simulink model "coupled_inductor_test"  (Simulink 7.4)
settings: Solver=ode45  StartTime=0.0  StopTime=10e-5  MaxStep=.001  RelTol=1e-4
StartFcn:
  | tic
StopFcn:
  | trun=toc
undefined symbols (not defined in the file or in its folder): Fs, magnitude
libraries: powerlib x16, dspindex x6, dsparch4 x5, dspsigops x3, dspsnks4 x2, dspbuff3 x2, dspxfrm3 x2, dsparch3 x2, dspmtrx3 x1, simulink x1
settings Model: Creator=Owner  LastModifiedBy=Dick
settings DataIOCC: SignalLoggingName=sigsOut
settings OptimizationCC: InlineInvariantSignals=on  InitFltsAndDblsToZero=on
settings DebuggingCC: SaveWithParameterizedLinksMsg=none  SignalResolutionControl=TryResolveAllWithWarning  SolverPrmCheckMsg=none  MultiTaskDSMMsg=warning  MultiTaskCondExecSysMsg=none  StrictBusMsg=None
settings HardwareCC: TargetUnknown=on
settings RTWCC: IncludeERTFirstTime=on
settings GRTTargetCC: TargetFcnLib=ansi_tfl_tmw.mat

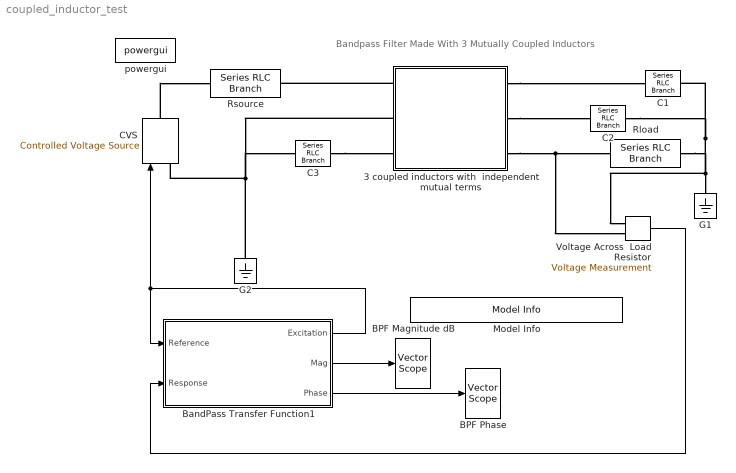
== system coupled_inductor_test ==
  note: Bandpass Filter Made With 3 Mutually Coupled Inductors
  3 coupled inductors with  independent mutual terms : Subsystem  mask{L1=1e-6, L2=1e-6, L3=1e-6, M12=0.1e-6, M23=0.1e-6, M13=1e-8}
      mask prompts: L1 "L1="; L2 "L2="; L3 "L3="; M12 "M12="; M23 "M23="; M13 "M13="
  BPF Magnitude dB : dspsnks4/Vector Scope  DialogController=dspdialog.VectorScope  DialogControllerArgs=DataTag0  ScopeProperties=on  Domain=Frequency  HorizSpan=1  DisplayProperties=off  AxisGrid=on  Memory=off  FrameNumber=on  AxisLegend=off  AxisZoom=off  OpenScopeAtSimStart=on  OpenScopeImmediately=off  FigPos=[38 401 372 236]  AxisProperties=off  XUnits=Hertz  XRange=[-Fs/2...Fs/2]  InheritXIncr=on  XIncr=2*Fs  XLabel=Time  XLimit=Auto  XMin=0  XMax=1  XStart=0  YUnits=dB  YLabel=dB  LineProperties=off  LineColors=[0 0 1]|[1 0 0]  XAxisParamsVer=6.9
      settings: YMin=-60  YMax=0
  BPF Phase : dspsnks4/Vector Scope  DialogController=dspdialog.VectorScope  DialogControllerArgs=DataTag1  ScopeProperties=on  Domain=Frequency  HorizSpan=1  DisplayProperties=off  AxisGrid=on  Memory=off  FrameNumber=on  AxisLegend=off  AxisZoom=off  OpenScopeAtSimStart=on  OpenScopeImmediately=off  FigPos=[37 115 372 236]  AxisProperties=off  XUnits=Hertz  XRange=[-Fs/2...Fs/2]  InheritXIncr=on  XIncr=2*Fs  XLabel=Time  XLimit=Auto  XMin=0  XMax=1  XStart=0  YUnits=Magnitude  YLabel=Degrees  LineProperties=off  LineColors=[0 0 1]|[1 0 0]  XAxisParamsVer=6.9
      settings: YMin=-253.502574206464  YMax=262.314910592616
  BandPass Transfer Function1 : Subsystem  Description=Spectrum Analyzer  mask{BW=40e6, Fc=100e6, NFFT=1024, Avg_fac=100}
      mask prompts: BW "Bandwidth"; Fc "Center Freq"; NFFT "FFT Length (power of 2)"; Avg_fac "Averaging Factor (>=1)"
  C1 : powerlib/Elements/Series RLC Branch  DialogController=POWERSYS.PowerSysDialog  PhysicalDomain=powersysdomain  SubClassName=unknown  LeftPortType=p1  RightPortType=p1  LConnTagsString=__new0  RConnTagsString=__new0  BranchType=C  Resistance=1.0  Inductance=1.0  SetiL0=off  InitialCurrent=0  Capacitance=2.5e-12  Setx0=off  InitialVoltage=0  Measurements=None
  C2 : powerlib/Elements/Series RLC Branch  DialogController=POWERSYS.PowerSysDialog  PhysicalDomain=powersysdomain  SubClassName=unknown  LeftPortType=p1  RightPortType=p1  LConnTagsString=__new0  RConnTagsString=__new0  BranchType=C  Resistance=1.0  Inductance=1.0  SetiL0=off  InitialCurrent=0  Capacitance=2.5e-12  Setx0=off  InitialVoltage=0  Measurements=None
  C3 : powerlib/Elements/Series RLC Branch  DialogController=POWERSYS.PowerSysDialog  PhysicalDomain=powersysdomain  SubClassName=unknown  LeftPortType=p1  RightPortType=p1  LConnTagsString=__new0  RConnTagsString=__new0  BranchType=C  Resistance=1.0  Inductance=1.0  SetiL0=off  InitialCurrent=0  Capacitance=2.5e-12  Setx0=off  InitialVoltage=0  Measurements=None
  CVS : powerlib/Electrical Sources/Controlled Voltage Source  Description=source block  DialogController=POWERSYS.PowerSysDialog  SystemSampleTime=-1  Initialize=on  Source_Type=AC  Amplitude=0  Phase=0  Frequency=0  Measurements=None
      settings: AttributesFormatString=\n
  G1 : powerlib/Elements/Ground  DialogController=POWERSYS.PowerSysDialog  PhysicalDomain=powersysdomain  SubClassName=unknown  LeftPortType=p1  RightPortType=p1  LConnTagsString=a
  G2 : powerlib/Elements/Ground  DialogController=POWERSYS.PowerSysDialog  PhysicalDomain=powersysdomain  SubClassName=unknown  LeftPortType=p1  RightPortType=p1  LConnTagsString=a
  Model Info : simulink/Model-Wide Utilities/Model Info  SystemSampleTime=-1  InitialBlockCM=None  BlockCM=None  Frame=on  DisplayStringWithTags=Copywrite 2005-2010 The MathWorks, Inc.  HorizontalTextAlignment=Center  LeftAlignmentValue=0.5  SourceBlockDiagram=coupled_inductor_test  TagMaxNumber=20
  Rload : powerlib/Elements/Series RLC Branch  DialogController=POWERSYS.PowerSysDialog  PhysicalDomain=powersysdomain  SubClassName=unknown  LeftPortType=p1  RightPortType=p1  LConnTagsString=__new0  RConnTagsString=__new0  BranchType=R  Resistance=50  Inductance=1.0  SetiL0=off  InitialCurrent=0  Capacitance=1.0  Setx0=off  InitialVoltage=0  Measurements=None
  Rsource : powerlib/Elements/Series RLC Branch  DialogController=POWERSYS.PowerSysDialog  PhysicalDomain=powersysdomain  SubClassName=unknown  LeftPortType=p1  RightPortType=p1  LConnTagsString=__new0  RConnTagsString=__new0  BranchType=R  Resistance=50  Inductance=1.0  SetiL0=off  InitialCurrent=0  Capacitance=1.0  Setx0=off  InitialVoltage=0  Measurements=None
  Voltage Across  Load Resistor : powerlib/Measurements/Voltage Measurement  Tag=PoWeRsYsTeMmEaSuReMeNt  DialogController=POWERSYS.PowerSysDialog  SystemSampleTime=-1  PhasorSimulation=off  OutputType=Magnitude  PSBequivalent=0
  powergui : powerlib/powergui  SystemSampleTime=-1  SimulationMode=Continuous  SampleTime=0  frequency=60  SPID=off  DisableSnubberDevices=off  DisableRonSwitches=off  DisableVfSwitches=off  SwTol=0  Interpol=off  frequencyindice=0  echomessages=off  HookPort=off  DisplayEquations=off  FunctionMessages=off  EnableUseOfTLC=off  x0status=blocks  RestoreLinks=warning  Frange=[0:2:500]  Ylog=off  Xlog=on  ShowGrid=off  save=off  variable=ZData  ZoomFFT=on  StartTime=0.0  cycles=1  DisplayStyle=1  fundamental=60  FreqAxis=off  MaxFrequency=1000  frequencyindicesteady=1  RmsSteady=1  display=off  Ts=0  methode=off
  wires:
  Voltage Across  Load Resistor/1 -> BandPass Transfer Function1/2(Response)
  BandPass Transfer Function1/1(Excitation) -> CVS/1, BandPass Transfer Function1/1(Reference)
  BandPass Transfer Function1/2(Mag) -> BPF Magnitude dB/1
  BandPass Transfer Function1/3(Phase) -> BPF Phase/1
  connections:
  3 coupled inductors with  independent mutual terms/LConn1 -- Rsource/RConn1
  CVS/RConn1 -- Rsource/LConn1
  C1/RConn1 -- C2/RConn1 -- Rload/RConn1 -- G1/LConn1 -- Voltage Across  Load Resistor/LConn1
  3 coupled inductors with  independent mutual terms/RConn3 -- Rload/LConn1 -- Voltage Across  Load Resistor/LConn2
  3 coupled inductors with  independent mutual terms/RConn2 -- C2/LConn1
  3 coupled inductors with  independent mutual terms/RConn1 -- C1/LConn1
  C3/RConn1 -- 3 coupled inductors with  independent mutual terms/LConn3
  G2/LConn1 -- 3 coupled inductors with  independent mutual terms/LConn2 -- C3/LConn1 -- CVS/LConn1

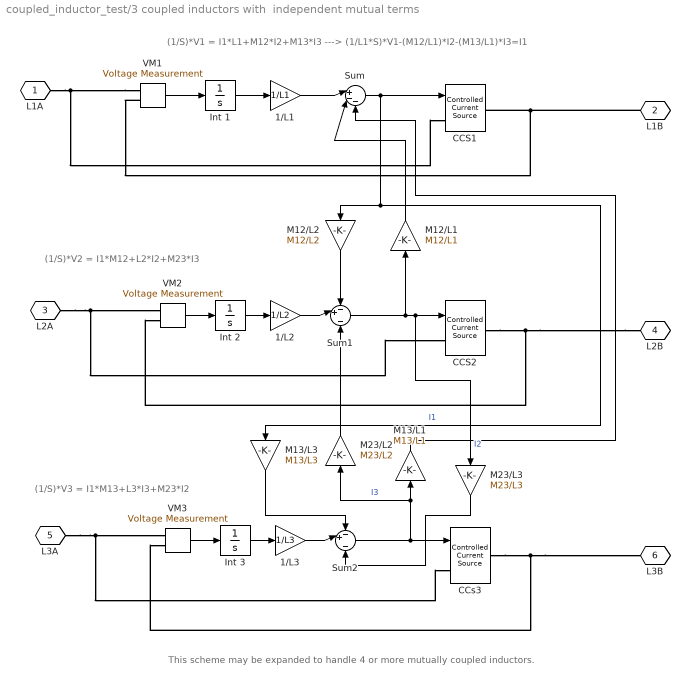
== system coupled_inductor_test/3 coupled inductors with  independent mutual terms ==
  note: (1/S)*V1 = I1*L1+M12*I2+M13*I3 ---> (1/L1*S)*V1-(M12/L1)*I2-(M13/L1)*I3=I1
  note: (1/S)*V2 = I1*M12+L2*I2+M23*I3
  note: (1/S)*V3 = I1*M13+L3*I3+M23*I2
  note: This scheme may be expanded to handle 4 or more mutually coupled inductors.
  1/L1 : Gain  Gain=1/L1  ParameterDataType=sfix(16)  ParameterScaling=2^0  OutDataType=sfix(16)  OutScaling=2^0  SaturateOnIntegerOverflow=on  OutDataTypeStr=Inherit: Same as input  ParamDataTypeStr=Inherit: Same as input
  1/L2 : Gain  Gain=1/L2  ParameterDataType=sfix(16)  ParameterScaling=2^0  OutDataType=sfix(16)  OutScaling=2^0  SaturateOnIntegerOverflow=on  OutDataTypeStr=Inherit: Same as input  ParamDataTypeStr=Inherit: Same as input
  1/L3 : Gain  Gain=1/L3  ParameterDataType=sfix(16)  ParameterScaling=2^0  OutDataType=sfix(16)  OutScaling=2^0  SaturateOnIntegerOverflow=on  OutDataTypeStr=Inherit: Same as input  ParamDataTypeStr=Inherit: Same as input
  CCS1 : powerlib/Electrical Sources/Controlled Current Source  Description=source block  DialogController=POWERSYS.PowerSysDialog  SystemSampleTime=-1  Initialize=off  Source_Type=AC  Amplitude=0  Phase=0  Frequency=0  Measurements=None
      settings: AttributesFormatString=\n
  CCS2 : powerlib/Electrical Sources/Controlled Current Source  Description=source block  DialogController=POWERSYS.PowerSysDialog  SystemSampleTime=-1  Initialize=off  Source_Type=AC  Amplitude=0  Phase=0  Frequency=0  Measurements=None
      settings: AttributesFormatString=\n
  CCs3 : powerlib/Electrical Sources/Controlled Current Source  Description=source block  DialogController=POWERSYS.PowerSysDialog  SystemSampleTime=-1  Initialize=off  Source_Type=AC  Amplitude=0  Phase=0  Frequency=0  Measurements=None
      settings: AttributesFormatString=\n
  Int 1 : Integrator
  Int 2 : Integrator
  Int 3 : Integrator
  M12/L1 : Gain  Gain=M12/L1  ParameterDataType=sfix(16)  ParameterScaling=2^0  OutDataType=sfix(16)  OutScaling=2^0  SaturateOnIntegerOverflow=on  OutDataTypeStr=Inherit: Same as input  ParamDataTypeStr=Inherit: Same as input
  M12/L2 : Gain  Gain=M12/L2  ParameterDataType=sfix(16)  ParameterScaling=2^0  OutDataType=sfix(16)  OutScaling=2^0  SaturateOnIntegerOverflow=on  OutDataTypeStr=Inherit: Same as input  ParamDataTypeStr=Inherit: Same as input
  M13/L1 : Gain  Gain=M13/L1  ParameterDataType=sfix(16)  ParameterScaling=2^0  OutDataType=sfix(16)  OutScaling=2^0  SaturateOnIntegerOverflow=on  OutDataTypeStr=Inherit: Same as input  ParamDataTypeStr=Inherit: Same as input
  M13/L3 : Gain  Gain=M13/L3  ParameterDataType=sfix(16)  ParameterScaling=2^0  OutDataType=sfix(16)  OutScaling=2^0  SaturateOnIntegerOverflow=on  OutDataTypeStr=Inherit: Same as input  ParamDataTypeStr=Inherit: Same as input
  M23/L2 : Gain  Gain=M23/L2  ParameterDataType=sfix(16)  ParameterScaling=2^0  OutDataType=sfix(16)  OutScaling=2^0  SaturateOnIntegerOverflow=on  OutDataTypeStr=Inherit: Same as input  ParamDataTypeStr=Inherit: Same as input
  M23/L3 : Gain  Gain=M23/L3  ParameterDataType=sfix(16)  ParameterScaling=2^0  OutDataType=sfix(16)  OutScaling=2^0  SaturateOnIntegerOverflow=on  OutDataTypeStr=Inherit: Same as input  ParamDataTypeStr=Inherit: Same as input
  Sum : Sum  Inputs=|+--  OutDataType=sfix(16)  OutScaling=2^0  SaturateOnIntegerOverflow=on
  Sum1 : Sum  Inputs=-+|-  OutDataType=sfix(16)  OutScaling=2^0  SaturateOnIntegerOverflow=on
  Sum2 : Sum  Inputs=-+|-  OutDataType=sfix(16)  OutScaling=2^0  SaturateOnIntegerOverflow=on
  VM1 : powerlib/Measurements/Voltage Measurement  Tag=PoWeRsYsTeMmEaSuReMeNt  DialogController=POWERSYS.PowerSysDialog  SystemSampleTime=-1  PhasorSimulation=off  OutputType=Magnitude  PSBequivalent=0
  VM2 : powerlib/Measurements/Voltage Measurement  Tag=PoWeRsYsTeMmEaSuReMeNt  DialogController=POWERSYS.PowerSysDialog  SystemSampleTime=-1  PhasorSimulation=off  OutputType=Magnitude  PSBequivalent=0
  VM3 : powerlib/Measurements/Voltage Measurement  Tag=PoWeRsYsTeMmEaSuReMeNt  DialogController=POWERSYS.PowerSysDialog  SystemSampleTime=-1  PhasorSimulation=off  OutputType=Magnitude  PSBequivalent=0
  L1A : PMIOPort  Tag=PMCPort  Port=1  Side=Left
  L1B : PMIOPort  Tag=PMCPort  Port=2  Side=Right
  L2A : PMIOPort  Tag=PMCPort  Port=3  Side=Left
  L2B : PMIOPort  Tag=PMCPort  Port=4  Side=Right
  L3A : PMIOPort  Tag=PMCPort  Port=5  Side=Left
  L3B : PMIOPort  Tag=PMCPort  Port=6  Side=Right
  wires:
  Int 1/1 -> 1/L1/1
  VM1/1 -> Int 1/1
  Int 2/1 -> 1/L2/1
  VM2/1 -> Int 2/1
  1/L1/1 -> Sum/1
  Sum/1 -> CCS1/1, M12/L2/1, M13/L3/1  "I1"
  Sum1/1 -> M12/L1/1, CCS2/1, M23/L3/1  "I2"
  1/L2/1 -> Sum1/2
  M12/L1/1 -> Sum/2
  M12/L2/1 -> Sum1/1
  Int 3/1 -> 1/L3/1
  VM3/1 -> Int 3/1
  Sum2/1 -> CCs3/1, M13/L1/1, M23/L2/1  "I3"
  1/L3/1 -> Sum2/2
  M13/L1/1 -> Sum/3
  M23/L2/1 -> Sum1/3
  M13/L3/1 -> Sum2/1
  M23/L3/1 -> Sum2/3
  connections:
  VM1/LConn1 -- L1A/RConn1 -- CCS1/LConn1
  VM1/LConn2 -- CCS1/RConn1 -- L1B/RConn1
  L2A/RConn1 -- VM2/LConn1 -- CCS2/LConn1
  L2B/RConn1 -- CCS2/RConn1 -- VM2/LConn2
  CCs3/LConn1 -- L3A/RConn1 -- VM3/LConn1
  VM3/LConn2 -- L3B/RConn1 -- CCs3/RConn1

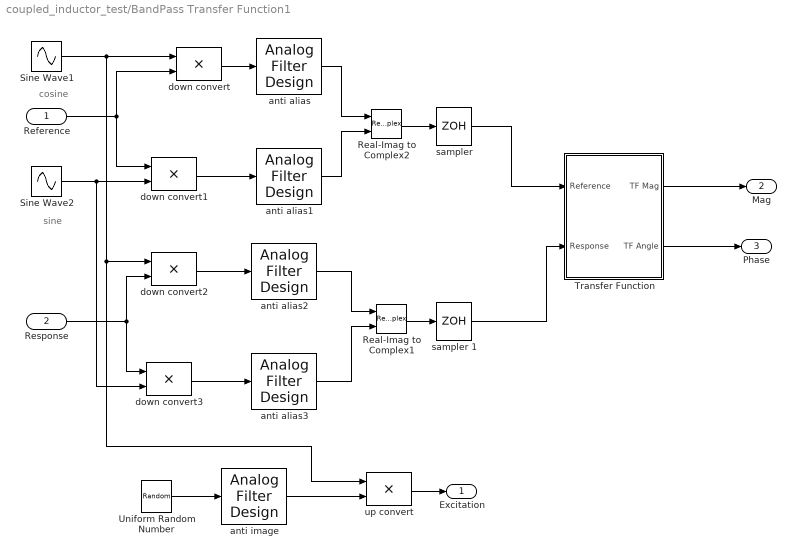
== system coupled_inductor_test/BandPass Transfer Function1 ==
  note: sine
  note: cosine
  Reference : Inport  OutDataType=sfix(16)  OutScaling=2^0
  Response : Inport  Port=2  OutDataType=sfix(16)  OutScaling=2^0
  Real-Imag to Complex1 : RealImagToComplex
  Real-Imag to Complex2 : RealImagToComplex
  Sine Wave1 : Sin  Amplitude=1  Bias=0  Frequency=2*pi*(Fc)  Phase=-pi/2  Samples=10  SampleTime=0  Offset=0
  Sine Wave2 : Sin  Amplitude=1  Bias=0  Frequency=2*pi*(Fc)  Phase=0  Samples=10  SampleTime=0  Offset=0
  "Transfer Function " : Subsystem  mask{NFFT=NFFT, Navg=Avg_fac, pcnt=100/1.28, unwrap_flag=on}
      mask prompts: NFFT "FFT length (power of 2):"; Navg "Spectral Averaging Factor (>=1):"; pcnt "Percentage of  Alias Free Data  (<=100)"; unwrap_flag "Unwrap Phase"
      mask Display: disp('Transfer Function \n Estimation (v2.0) ')
  Uniform Random Number : UniformRandomNumber  SampleTime=1/(2.56*BW)
  anti alias{,1..3} (4 alike) : dsparch4/Analog Filter Design  method=Elliptic  filttype=Lowpass  N=8  Wlo=BW*pi  Whi=80  Rp=2  Rs=100
  anti image : dsparch4/Analog Filter Design  method=Elliptic  filttype=Lowpass  N=9  Wlo=BW*pi  Whi=80  Rp=2  Rs=100
  down convert{,1..3} (4 alike) : Product  OutDataType=sfix(16)  OutScaling=2^0  SaturateOnIntegerOverflow=on  InputSameDT=on  OutDataTypeStr=Inherit: Same as first input
  "sampler " : ZeroOrderHold  SampleTime=1/(1.28*BW)
  sampler 1 : ZeroOrderHold  SampleTime=1/(1.28*BW)
  up convert : Product  OutDataType=sfix(16)  OutScaling=2^0  SaturateOnIntegerOverflow=on  InputSameDT=on  OutDataTypeStr=Inherit: Same as first input
  Excitation : Outport  OutDataType=sfix(16)  OutScaling=2^0
  Mag : Outport  Port=2  OutDataType=sfix(16)  OutScaling=2^0
  Phase : Outport  Port=3  OutDataType=sfix(16)  OutScaling=2^0
  wires:
  anti image/1 -> up convert/2
  down convert1/1 -> anti alias1/1
  sampler 1/1 -> "Transfer Function "/2(Response)
  "sampler "/1 -> "Transfer Function "/1(Reference)
  Real-Imag to Complex2/1 -> "sampler "/1
  anti alias1/1 -> Real-Imag to Complex2/2
  anti alias/1 -> Real-Imag to Complex2/1
  "Transfer Function "/2(TF Angle) -> Phase/1
  "Transfer Function "/1(TF Mag) -> Mag/1
  up convert/1 -> Excitation/1
  Uniform Random Number/1 -> anti image/1
  Real-Imag to Complex1/1 -> sampler 1/1
  down convert3/1 -> anti alias3/1
  anti alias3/1 -> Real-Imag to Complex1/2
  anti alias2/1 -> Real-Imag to Complex1/1
  down convert2/1 -> anti alias2/1
  Response/1 -> down convert2/2, down convert3/1
  Sine Wave2/1 -> down convert3/2, down convert1/2
  Sine Wave1/1 -> up convert/1, down convert2/1, down convert/1
  down convert/1 -> anti alias/1
  Reference/1 -> down convert1/1, down convert/2

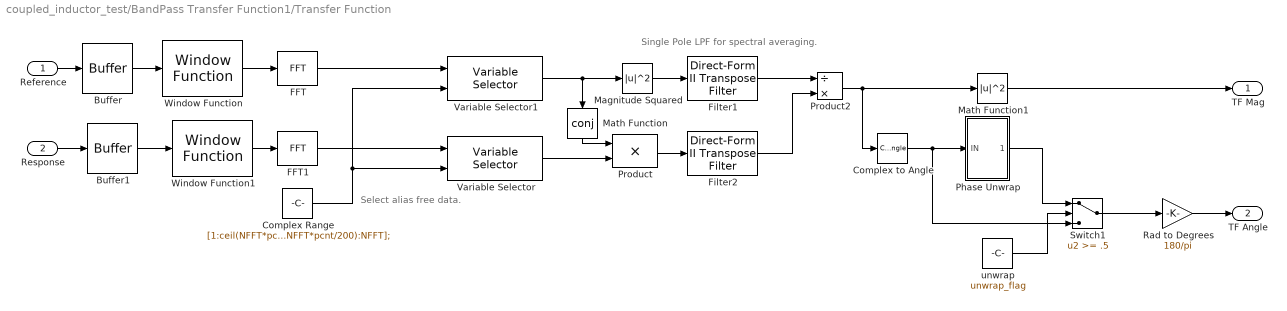
== system coupled_inductor_test/BandPass Transfer Function1/Transfer Function  ==
  note: Select alias free data.
  note: Single Pole LPF for spectral averaging.
  Reference : Inport  OutDataType=sfix(16)  OutScaling=2^0
  Response : Inport  Port=2  OutDataType=sfix(16)  OutScaling=2^0
  Buffer : dspbuff3/Buffer  N=NFFT  V=0  ic=0
  Buffer1 : dspbuff3/Buffer  N=NFFT  V=0  ic=0
  Complex Range : Constant  Value=[1:ceil(NFFT*pcnt/200),ceil(1+NFFT-NFFT*pcnt/200):NFFT];  OutDataType=sfix(16)  OutScaling=2^0
  Complex to Angle : ComplexToMagnitudeAngle  Output=Angle
  FFT : dspxfrm3/FFT  DialogController=dspDDGCreate  DialogControllerArgs=DataTag2  CompMethod=Table lookup  TableOpt=NEW  TableOptActive=Speed  BitRevOrder=off  InheritFFTLength=on  FFTLength=64  SkipNorm=on  firstCoeffMode=Specify word length  firstCoeffWordLength=16  firstCoeffFracLength=15  roundingMode=Floor  overflowMode=off
  FFT1 : dspxfrm3/FFT  DialogController=dspDDGCreate  DialogControllerArgs=DataTag3  CompMethod=Table lookup  TableOpt=NEW  TableOptActive=Speed  BitRevOrder=off  InheritFFTLength=on  FFTLength=64  SkipNorm=on  firstCoeffMode=User-defined  firstCoeffWordLength=16  firstCoeffFracLength=15  roundingMode=Floor  overflowMode=off
  Filter1 : dsparch3/Direct-Form II Transpose Filter  num=1  den=[Navg -(Navg-1)]  ic=eps
  Filter2 : dsparch3/Direct-Form II Transpose Filter  num=1  den=[Navg -(Navg-1)]  ic=eps
  Magnitude Squared : Math  Operator=magnitude^2  OutDataType=sfix(16)  OutScaling=2^0  SaturateOnIntegerOverflow=on
  Math Function : Math  Operator=conj  OutDataType=sfix(16)  OutScaling=2^0  SaturateOnIntegerOverflow=on
  Math Function1 : Math  Operator=magnitude^2  OutDataType=sfix(16)  OutScaling=2^0  SaturateOnIntegerOverflow=on
  Phase Unwrap : Subsystem
  Product : Product  OutDataType=sfix(16)  OutScaling=2^0  SaturateOnIntegerOverflow=on  InputSameDT=on  OutDataTypeStr=Inherit: Same as first input
  Product2 : Product  Inputs=/*  OutDataType=sfix(16)  OutScaling=2^0  SaturateOnIntegerOverflow=on  InputSameDT=on  OutDataTypeStr=Inherit: Same as first input
  Rad to Degrees : Gain  Gain=180/pi  ParameterDataType=sfix(16)  ParameterScaling=2^0  OutDataType=sfix(16)  OutScaling=2^0
  Switch1 : Switch  Threshold=.5
  Variable Selector : dspindex/Variable Selector  NumInputs=1  rowsOrCols=Rows  IdxMode=Variable  Elements=[1 3]  ZerOneIdxMode=One-based  errmode=Clip Index  FillMode=on  FillValues=0
  Variable Selector1 : dspindex/Variable Selector  NumInputs=1  rowsOrCols=Rows  IdxMode=Variable  Elements=[1 3]  ZerOneIdxMode=One-based  errmode=Clip Index  FillMode=on  FillValues=0
  Window Function : dspsigops/Window Function  DialogController=dspDDGCreate  DialogControllerArgs=DataTag5  winmode=Apply window to input  wintype=Hann  sampmode=Continuous  samptime=1  N=64  Rs=50  beta=10  winsamp=Periodic  UserWindow=hamming  OptParams=off  UserParams={'symmetric'}  dataType=double  isSigned=on  wordLen=16  udDataType=sfix(16)  fracBitsMode=Best precision  numFracBits=15  roundingMode=Floor  overflowMode=off  numSidelobes=4  sidelobeLevel=-30
  Window Function1 : dspsigops/Window Function  DialogController=dspDDGCreate  DialogControllerArgs=DataTag6  winmode=Apply window to input  wintype=Hann  sampmode=Continuous  samptime=1  N=64  Rs=50  beta=10  winsamp=Periodic  UserWindow=hamming  OptParams=off  UserParams={'symmetric'}  dataType=double  isSigned=on  wordLen=16  udDataType=sfix(16)  fracBitsMode=Best precision  numFracBits=15  roundingMode=Floor  overflowMode=off  numSidelobes=4  sidelobeLevel=-30
  unwrap : Constant  Value=unwrap_flag  OutDataType=sfix(16)  OutScaling=2^0
  TF Mag : Outport  OutDataType=sfix(16)  OutScaling=2^0
  TF Angle : Outport  Port=2  OutDataType=sfix(16)  OutScaling=2^0
  wires:
  Phase Unwrap/1(Out1) -> Switch1/1
  unwrap/1 -> Switch1/2
  Switch1/1 -> Rad to Degrees/1
  Variable Selector1/1 -> Math Function/1, Magnitude Squared/1
  Variable Selector/1 -> Product/2
  Product2/1 -> Math Function1/1, Complex to Angle/1
  Buffer1/1 -> Window Function1/1
  Buffer/1 -> Window Function/1
  Filter2/1 -> Product2/2
  Filter1/1 -> Product2/1
  Window Function1/1 -> FFT1/1
  Window Function/1 -> FFT/1
  Math Function1/1 -> TF Mag/1
  FFT/1 -> Variable Selector1/1
  Magnitude Squared/1 -> Filter1/1
  Math Function/1 -> Product/1
  FFT1/1 -> Variable Selector/1
  Product/1 -> Filter2/1
  Reference/1 -> Buffer/1
  Response/1 -> Buffer1/1
  Rad to Degrees/1 -> TF Angle/1
  Complex to Angle/1 -> Phase Unwrap/1(IN), Switch1/3
  Complex Range/1 -> Variable Selector1/2, Variable Selector/2

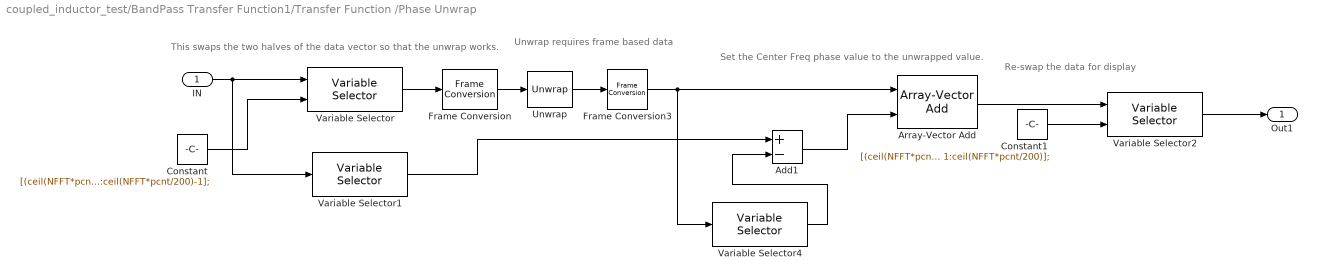
== system coupled_inductor_test/BandPass Transfer Function1/Transfer Function /Phase Unwrap ==
  note: Unwrap requires frame based data
  note: Re-swap the data for display
  note: Set the Center Freq phase value to the unwrapped value.
  note: This swaps the two halves of the data vector
      | so that the unwrap works.
  IN : Inport  OutDataType=sfix(16)  OutScaling=2^0
  Add1 : Sum  Inputs=+-  OutDataType=sfix(16)  OutScaling=2^-10
  Array-Vector Add : dspmtrx3/Array-Vector Add  DialogController=dspDDGCreate  DialogControllerArgs=DataTag4  Dimension=2  V_Source=Input port  V_VectFromMask=[0.5 0.25]  firstCoeffDataTypeStr=Inherit: Same word length as input  firstCoeffLastDataTypeStr=Inherit: Same word length as input  firstCoeffMin=[]  firstCoeffMax=[]  outputDataTypeStr=Inherit: Same as accumulator  outputLastDataTypeStr=Inherit: Same as accumulator  outputMin=[]  outputMax=[]  roundingMode=Floor  overflowMode=off
  Constant : Constant  Value=[(ceil(NFFT*pcnt/200)):ceil(NFFT*pcnt/100) 1:ceil(NFFT*pcnt/200)-1];  OutDataType=sfix(16)  OutScaling=2^0
  Constant1 : Constant  Value=[(ceil(NFFT*pcnt/200)+1):ceil(NFFT*pcnt/100) 1:ceil(NFFT*pcnt/200)];  OutDataType=sfix(16)  OutScaling=2^0
  Frame Conversion : FrameConversion
  Frame Conversion3 : FrameConversion  OutFrame=Sample-based
  Unwrap : dspsigops/Unwrap  running=on  tol=pi
  Variable Selector : dspindex/Variable Selector  NumInputs=1  rowsOrCols=Rows  IdxMode=Variable  Elements=[1 3]  ZerOneIdxMode=One-based  errmode=Clip Index  FillMode=on  FillValues=0
  Variable Selector1 : dspindex/Variable Selector  NumInputs=1  rowsOrCols=Rows  IdxMode=Fixed  Elements=[1]  ZerOneIdxMode=One-based  errmode=Clip Index  FillMode=on  FillValues=0
  Variable Selector2 : dspindex/Variable Selector  NumInputs=1  rowsOrCols=Rows  IdxMode=Variable  Elements=[1 3]  ZerOneIdxMode=One-based  errmode=Clip Index  FillMode=on  FillValues=0
  Variable Selector4 : dspindex/Variable Selector  NumInputs=1  rowsOrCols=Rows  IdxMode=Fixed  Elements=length([(ceil(NFFT*pcnt/200)+1):ceil(NFFT*pcnt/100) 1:ceil(NFFT*pcnt/200)] )/2+1  ZerOneIdxMode=One-based  errmode=Clip Index  FillMode=on  FillValues=0
  Out1 : Outport  OutDataType=sfix(16)  OutScaling=2^0
  wires:
  Array-Vector Add/1 -> Variable Selector2/1
  Add1/1 -> Array-Vector Add/2
  Frame Conversion3/1 -> Array-Vector Add/1, Variable Selector4/1
  Constant1/1 -> Variable Selector2/2
  Variable Selector4/1 -> Add1/2
  Unwrap/1 -> Frame Conversion3/1
  Variable Selector1/1 -> Add1/1
  Variable Selector/1 -> Frame Conversion/1
  Constant/1 -> Variable Selector/2
  IN/1 -> Variable Selector1/1, Variable Selector/1
  Variable Selector2/1 -> Out1/1
  Frame Conversion/1 -> Unwrap/1
